simulink model "mission_planner_test"  (R2015a)
settings: Solver=ode45  StartTime=0.0  StopTime=10.0  RelTol=1e-3
libraries: robotlib x10
settings Model: Creator=Kelan  LastModifiedBy=Kelan

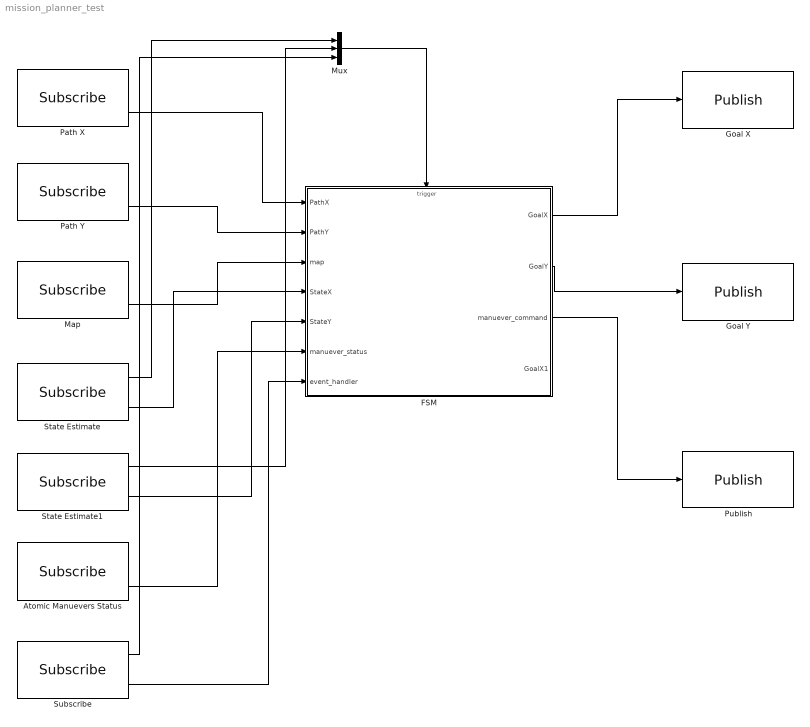
== system mission_planner_test ==
  Atomic Manuevers Status : robotlib/Subscribe  SourceLibraryInfo=This block requires Robotics System Toolbox  topicSource=Specify your own  topic=/manuevers_status  messageType=std_msgs/Bool  sampleTime=-1  messageQueueLength=1
  FSM : Stateflow chart  TreatAsAtomicUnit=on
  Goal X : robotlib/Publish  SourceLibraryInfo=This block requires Robotics System Toolbox  topicSource=Specify your own  topic=/GoalX  messageType=std_msgs/Int16  messageQueueLength=1
  Goal Y : robotlib/Publish  SourceLibraryInfo=This block requires Robotics System Toolbox  topicSource=Specify your own  topic=/GoalY  messageType=std_msgs/Int16  messageQueueLength=1
  Map : robotlib/Subscribe  SourceLibraryInfo=This block requires Robotics System Toolbox  topicSource=Specify your own  topic=/map  messageType=nav_msgs/OccupancyGrid  sampleTime=-1  messageQueueLength=1
  Mux : Mux  Inputs=3
  Path X : robotlib/Subscribe  SourceLibraryInfo=This block requires Robotics System Toolbox  topicSource=Specify your own  topic=/pathX  messageType=std_msgs/Int16MultiArray  sampleTime=-1  messageQueueLength=1
  Path Y : robotlib/Subscribe  SourceLibraryInfo=This block requires Robotics System Toolbox  topicSource=Specify your own  topic=/pathY  messageType=std_msgs/Int16MultiArray  sampleTime=-1  messageQueueLength=1
  Publish : robotlib/Publish  SourceLibraryInfo=This block requires Robotics System Toolbox  topicSource=Specify your own  topic=/manuever_command  messageType=std_msgs/Char  messageQueueLength=1
  State Estimate : robotlib/Subscribe  SourceLibraryInfo=This block requires Robotics System Toolbox  topicSource=Specify your own  topic=/stateX  messageType=std_msgs/Empty  sampleTime=-1  messageQueueLength=1
  State Estimate1 : robotlib/Subscribe  SourceLibraryInfo=This block requires Robotics System Toolbox  topicSource=Specify your own  topic=/stateY  messageType=std_msgs/Empty  sampleTime=-1  messageQueueLength=1
  Subscribe : robotlib/Subscribe  SourceLibraryInfo=This block requires Robotics System Toolbox  topicSource=Specify your own  topic=/event_handler  messageType=std_msgs/Empty  sampleTime=-1  messageQueueLength=1
  wires:
  FSM/1(GoalX) -> Goal X/1
  FSM/2(GoalY) -> Goal Y/1
  FSM/3(manuever_command) -> Publish/1
  Atomic Manuevers Status/2 -> FSM/6(manuever_status)
  State Estimate/2 -> FSM/4(StateX)
  Map/2 -> FSM/3(map)
  Path Y/2 -> FSM/2(PathY)
  Path X/2 -> FSM/1(PathX)
  Mux/1 -> FSM/Trigger
  State Estimate/1 -> Mux/1
  State Estimate1/1 -> Mux/2
  State Estimate1/2 -> FSM/5(StateY)
  Subscribe/1 -> Mux/3
  Subscribe/2 -> FSM/7(event_handler)

== stateflow chart mission_planner_test/FSM ==
  state Initialization
  state Preliminary
    (default) -> (junction 209) : % Red Buoy 1
    (junction 209) -> (junction 208) [order 1] : [event = red_Buoy]
    (junction 209) -> (junction 210) [order 2]
    (junction 208) -> (junction 207) : {red1 = [posX, posY];}
    (junction 207) -> (junction 210)
    (junction 210) -> (junction 220) : % Green Buoy 1
    (junction 220) -> (junction 219) [order 1] : [event = green_Buoy]
    (junction 220) -> (junction 221) [order 2]
    (junction 219) -> (junction 218) : {green1 = [posX, posY];}
    (junction 218) -> (junction 221)
    (junction 221) -> (junction 234) : % End Buoy Search
    (junction 234) -> (junction 231)
    (junction 231) -> (junction 233) [order 1] : [event = 0;]
    (junction 233) -> (junction 230) : {GoalX = (red1(1)+green1(1))/2; GoalY=StateY+5;}
    (junction 230) -> (junction 231)
    (junction 231) -> (junction 245) [order 2] : % Red Buoy 2
    (junction 245) -> (junction 244) [order 1] : [event = red_Buoy]
    (junction 245) -> (junction 246) [order 2]
    (junction 244) -> (junction 243) : {red2 = [posX, posY];}
    (junction 243) -> (junction 246)
    (junction 246) -> (junction 256) : % Green Buoy 2
    (junction 256) -> (junction 255) [order 1] : [event = green_Buoy]
    (junction 256) -> (junction 257) [order 2]
    (junction 255) -> (junction 254) : {green2 = [posX, posY];}
    (junction 254) -> (junction 257)
    (junction 257) -> (junction 253)
  state Survey [group]
    (junction 123) -> (junction 125) : {loop=0}
    (junction 125) -> (junction 124) [order 1] : [detected=0]
    (junction 124) -> (junction 104) : {GoalY = StateY+10;}
    (junction 105) -> (junction 125) [order 1] : {loop=loop+1}
    (default) -> (junction 125)
    (junction 125) -> (junction 120) [order 2]
    (junction 104) -> (junction 105) : {index=0;}
    (junction 105) -> (junction 111) [order 2] : [(detected=0)&&(index<12)]
    (junction 118) -> (junction 105) : {index=index+1;}
    (junction 111) -> (junction 110) [order 1] : [loop%2=0]
    (junction 111) -> (junction 112) [order 2] : {GoalX = StateX - 10;}
    (junction 110) -> (junction 119) : {GoalX = StateX + 10;}
    (junction 119) -> (junction 112)
    (junction 112) -> (junction 118)
  state Undock
    entry:
    busy=1;
    motion = undock();
  state Scan
    entry:
    busy=1;
    scan=[x,y];
  state Buoy
    entry:
    busy = 1;
    motion = [x, y, r, psi_in, psi_out];
  state Dock
    entry:
    busy=1;
    motion = dock();
  state Hold [group]
    (junction 152) -> (junction 151)
    (junction 151) -> (junction 150) : {GoalX = StateX;
        | GoalY = StateY;
        | manuever_command = 'h'}
    (junction 150) -> (junction 152) : [detected = 0]
  Initialization -> ? [order 4294967295] : {detected=1}
  (default) -> Initialization
  Initialization -> (junction 123) [order 1] : {manuever_status = 1}
  (junction 120) -> (junction 152) : [detected=0]
  Preliminary -> Hold
  data: PathX input; PathY input; map input; StateX input; StateY input; manuever_status input; GoalX output; GoalY output; manuever_command output; event_handler input; green1 local int16; green2 local int16; red1 local int16; red2 local int16; GoalX1 output
  events: detected input RISING_EDGE_EVENT; event input RISING_EDGE_EVENT
